simulink model "YawAngle_controller_test"  (R2018a)
settings: Solver=VariableStepAuto  StartTime=0.0  StopTime=15  RelTol=1e-3
settings Model: Creator=梁鑫  LastModifiedBy=梁鑫

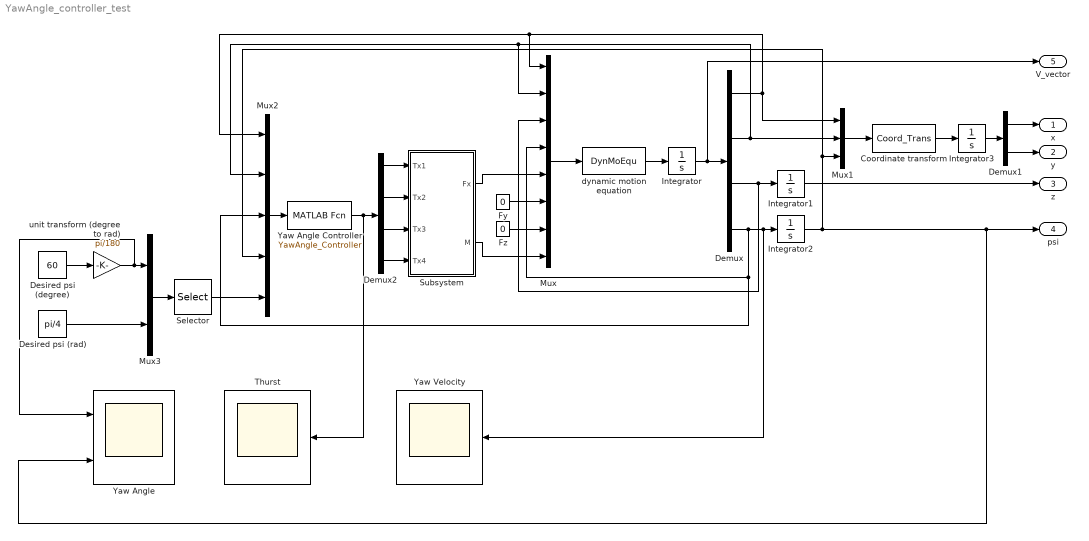
== system YawAngle_controller_test ==
  Coordinate transform : MATLABFcn  MATLABFcn=Coord_Trans  OutputDimensions=2
  Demux : Demux
  Demux1 : Demux  Outputs=2
  Demux2 : Demux
  Desired psi (degree) : Constant  Value=60
  Desired psi (rad) : Constant  Value=pi/4
  Fy : Constant  Value=0
  Fz : Constant  Value=0
  Integrator{,1..3} (4 alike) : Integrator
  Mux : Mux  Inputs=8
  Mux1 : Mux  Inputs=3
  Mux2 : Mux  Inputs=5
  Mux3 : Mux  Inputs=2
  Selector : Selector  InputPortWidth=2  IndexOptions=Index vector (dialog)  Indices=1  OutputSizes=1
  Subsystem : Subsystem
  Thurst : Scope
  Yaw Angle : Scope  NumInputPorts=2
  Yaw Angle Controller : MATLABFcn  MATLABFcn=YawAngle_Controller  OutputDimensions=4
  Yaw Velocity : Scope
  dynamic motion equation : MATLABFcn  MATLABFcn=DynMoEqu  OutputDimensions=4
  unit transform (degree to rad) : Gain  Gain=pi/180
  x : Outport
  y : Outport  Port=2
  z : Outport  Port=3
  psi : Outport  Port=4
  V_vector : Outport  Port=5
  wires:
  Mux/1 -> dynamic motion equation/1
  Mux1/1 -> Coordinate transform/1
  Fz/1 -> Mux/7
  Integrator/1 -> Demux/1, V_vector/1
  Demux/1 -> Mux1/1, Mux2/1, Mux/1
  Coordinate transform/1 -> Integrator3/1
  Demux1/2 -> y/1
  Demux/3 -> Mux/3, Integrator1/1
  Demux/4 -> Mux2/3, Mux/4, Yaw Velocity/1, Integrator2/1
  Demux1/1 -> x/1
  Integrator2/1 -> Yaw Angle/2, psi/1, Mux2/4, Mux1/3
  Integrator3/1 -> Demux1/1
  Integrator1/1 -> z/1
  Demux/2 -> Mux2/2, Mux/2, Mux1/2
  dynamic motion equation/1 -> Integrator/1
  Fy/1 -> Mux/6
  Mux2/1 -> Yaw Angle Controller/1
  Desired psi (degree)/1 -> unit transform (degree to rad)/1
  Yaw Angle Controller/1 -> Thurst/1, Demux2/1
  unit transform (degree to rad)/1 -> Yaw Angle/1, Mux3/1
  Desired psi (rad)/1 -> Mux3/2
  Mux3/1 -> Selector/1
  Selector/1 -> Mux2/5
  Demux2/1 -> Subsystem/1(Tx1)
  Demux2/2 -> Subsystem/2(Tx2)
  Demux2/3 -> Subsystem/3(Tx3)
  Demux2/4 -> Subsystem/4(Tx4)
  Subsystem/1(Fx) -> Mux/5
  Subsystem/2(M) -> Mux/8

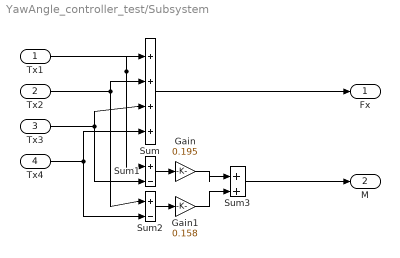
== system YawAngle_controller_test/Subsystem ==
  Tx1 : Inport
  Tx2 : Inport  Port=2
  Tx3 : Inport  Port=3
  Tx4 : Inport  Port=4
  Gain : Gain  Gain=0.195
  Gain1 : Gain  Gain=0.158
  Sum : Sum  Inputs=|++++
  Sum1 : Sum  Inputs=|+-
  Sum2 : Sum  Inputs=|+-
  Sum3 : Sum  Inputs=|++
  Fx : Outport
  M : Outport  Port=2
  wires:
  Tx1/1 -> Sum1/1, Sum/1
  Sum1/1 -> Gain/1
  Gain/1 -> Sum3/1
  Gain1/1 -> Sum3/2
  Tx2/1 -> Sum2/1, Sum/2
  Tx3/1 -> Sum1/2, Sum/3
  Tx4/1 -> Sum2/2, Sum/4
  Sum2/1 -> Gain1/1
  Sum/1 -> Fx/1
  Sum3/1 -> M/1
